simulink model "ManipRoboticoTraiettoriaSpazioGiunti"  (R2025b)
settings: Solver=VariableStepAuto  StartTime=0.0  StopTime=10  RelTol=1e-3
values from neighbouring files (symbols this model uses):
  Kd = [15; 15]    [main.m]
  Kp = [20; 20]    [main.m]
settings Model: Creator=arman  LastModifiedBy=arman

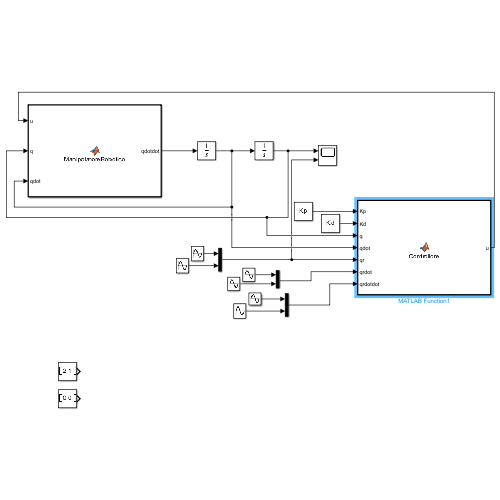
[thumbnail: Simulink's stored preview of the top-level diagram]
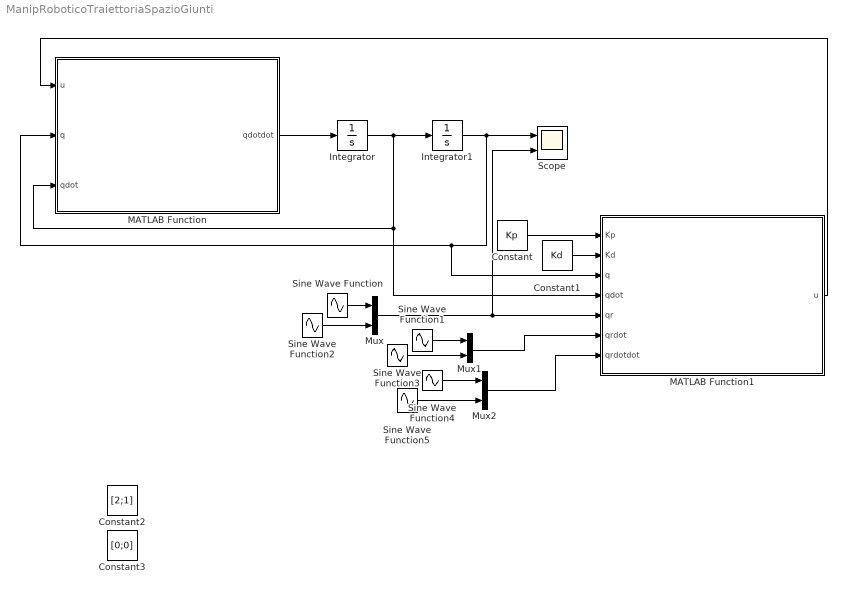
== system ManipRoboticoTraiettoriaSpazioGiunti ==
  Constant : Constant  Value=Kp
  Constant1 : Constant  Value=Kd
  Constant2 : Constant  Value=[2;1]
  Constant3 : Constant  Value=[0;0]
  Integrator : Integrator  InitialCondition=[0;0]
  Integrator1 : Integrator  InitialCondition=[0;0]
  MATLAB Function : MATLAB Function  TreatAsAtomicUnit=on
  MATLAB Function1 : MATLAB Function  TreatAsAtomicUnit=on
  Mux : Mux  Inputs=2
  Mux1 : Mux  Inputs=2
  Mux2 : Mux  Inputs=2
  Scope : Scope  NumInputPorts=2
      settings: ActiveDisplayYMinimum=-5.4938580572582376  ActiveDisplayYMaximum=2.8316295939504461
  Sine Wave Function : Sin  SampleTime=0
  Sine Wave Function1 : Sin  Phase=pi/2  SampleTime=0
  Sine Wave Function2 : Sin  Amplitude=2  SampleTime=0
  Sine Wave Function3 : Sin  Amplitude=2  Phase=pi/2  SampleTime=0
  Sine Wave Function4 : Sin  Amplitude=-1  SampleTime=0
  Sine Wave Function5 : Sin  Amplitude=-2  SampleTime=0
  wires:
  MATLAB Function/1(qdotdot) -> Integrator/1
  Integrator/1 -> MATLAB Function1/4(qdot), MATLAB Function/3(qdot), Integrator1/1
  Integrator1/1 -> MATLAB Function1/3(q), MATLAB Function/2(q), Scope/1
  Constant/1 -> MATLAB Function1/1(Kp)
  Constant1/1 -> MATLAB Function1/2(Kd)
  MATLAB Function1/1(u) -> MATLAB Function/1(u)
  Sine Wave Function/1 -> Mux/1
  Sine Wave Function2/1 -> Mux/2
  Mux/1 -> MATLAB Function1/5(qr), Scope/2
  Sine Wave Function1/1 -> Mux1/1
  Sine Wave Function3/1 -> Mux1/2
  Mux1/1 -> MATLAB Function1/6(qrdot)
  Sine Wave Function5/1 -> Mux2/2
  Sine Wave Function4/1 -> Mux2/1
  Mux2/1 -> MATLAB Function1/7(qrdotdot)

== matlab function ManipRoboticoTraiettoriaSpazioGiunti/MATLAB Function1 ==
  data: Kp input; Kd input; u output; q input; qdot input; qr input; qrdot input; qrdotdot input
function u = Controllore(Kp,Kd,q,qdot,qr,qrdot,qrdotdot)
e = q - qr;
edot = qdot - qrdot;
[B, C, g, F] = calculateMatrixRobotRR(q,qdot);
u = B*qrdotdot + C*qrdot + g  - Kp.*e - Kd.*edot;

== matlab function ManipRoboticoTraiettoriaSpazioGiunti/MATLAB Function ==
  data: u input; q input; qdotdot output; qdot input
function qdotdot = ManipolatoreRobotico(u,q,qdot)
[B, C, g, F] = calculateMatrixRobotRR(q,qdot);
qdotdot = B \ (u - (C * qdot) - g - F);
